simulink model "derivative_approx_filter"  (R2021a)
settings: Solver=ode1  StartTime=0.0  StopTime=10.0  FixedStep=Ts  MaxStep=1e-3  RelTol=1e-3
values from neighbouring files (symbols this model uses):
  wn = 100    [params.m]
  z = 0.7    [params.m]
undefined symbols (not defined in the file or in its folder): Noise
libraries: simulink x1
settings Model: Creator=perruquetti  LastModifiedBy=perruquetti

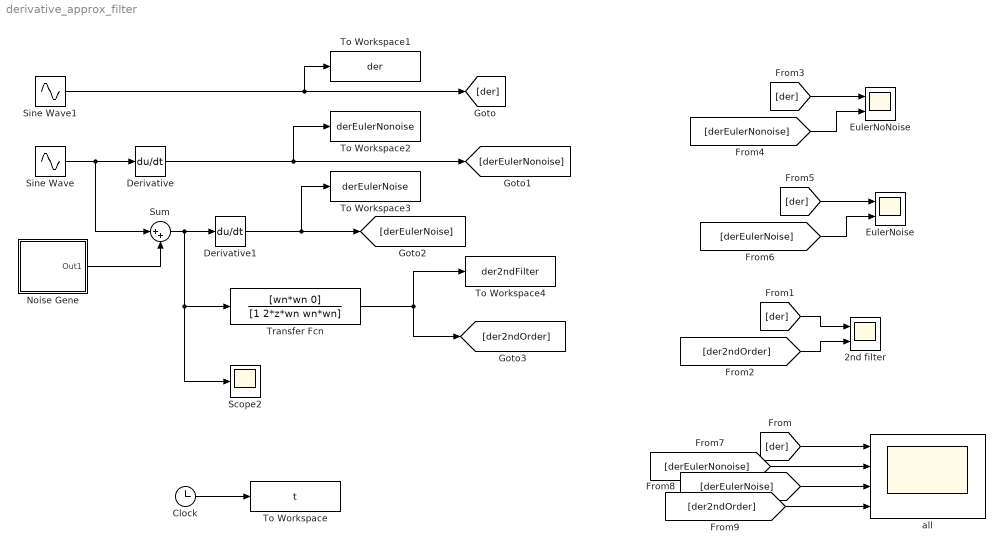
== system derivative_approx_filter ==
  2nd filter : Scope  NumInputPorts=2
  Clock : Clock
  Derivative : Derivative
  Derivative1 : Derivative
  EulerNoNoise : Scope  NumInputPorts=2
  EulerNoise : Scope  NumInputPorts=2
  Noise Gene : Subsystem
  Scope2 : Scope
  Sine Wave : Sin  Frequency=10  SampleTime=0
  Sine Wave1 : Sin  Amplitude=10  Frequency=10  Phase=90  SampleTime=0
  Sum : Sum  Inputs=|++
  To Workspace : ToWorkspace  VariableName=t  SampleTime=-1
  To Workspace1 : ToWorkspace  VariableName=der  SampleTime=-1
  To Workspace2 : ToWorkspace  VariableName=derEulerNonoise  SampleTime=-1
  To Workspace3 : ToWorkspace  VariableName=derEulerNoise  SampleTime=-1
  To Workspace4 : ToWorkspace  VariableName=der2ndFilter  SampleTime=-1
  Transfer Fcn : TransferFcn  Numerator=[wn*wn 0]  Denominator=[1 2*z*wn wn*wn]
  all : Scope  NumInputPorts=4
  wires:
  Sine Wave/1 -> Sum/1, Derivative/1
  Noise Gene/1(Out1) -> Sum/2
  Sum/1 -> Transfer Fcn/1, Scope2/1, Derivative1/1
  Sine Wave1/1 -> To Workspace1/1, [der]
  Derivative/1 -> To Workspace2/1, [derEulerNonoise]
  Derivative1/1 -> [derEulerNoise], To Workspace3/1
  Clock/1 -> To Workspace/1
  [der] -> all/1
  Transfer Fcn/1 -> [der2ndOrder], To Workspace4/1
  [der] -> 2nd filter/1
  [der2ndOrder] -> 2nd filter/2
  [der] -> EulerNoNoise/1
  [derEulerNonoise] -> EulerNoNoise/2
  [der] -> EulerNoise/1
  [derEulerNoise] -> EulerNoise/2
  [derEulerNonoise] -> all/2
  [derEulerNoise] -> all/3
  [der2ndOrder] -> all/4

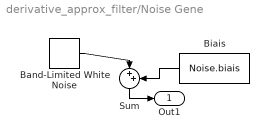
== system derivative_approx_filter/Noise Gene ==
  Band-Limited White Noise : simulink/Sources/Band-Limited White Noise  Cov=Noise.power  Ts=Noise.sampling  seed=Noise.seed
  Biais : Constant  Value=Noise.biais
  Sum : Sum  Inputs=|++
  Out1 : Outport
  wires:
  Sum/1 -> Out1/1
  Biais/1 -> Sum/2
  Band-Limited White Noise/1 -> Sum/1
